simulink model "encode_decode_withAlarms_correction1"  (R2022a)
settings: Solver=VariableStepAuto  StartTime=0.0  StopTime=200  RelTol=1e-3
libraries: simulink x7, spsSampleandHoldLib x2
settings Model: Creator=mluser  LastModifiedBy=mluser
settings ModelReferenceCC: EnableRefExpFcnMdlSchedulingChecks=off
settings RTWCC: Description=Generic Real-Time Target

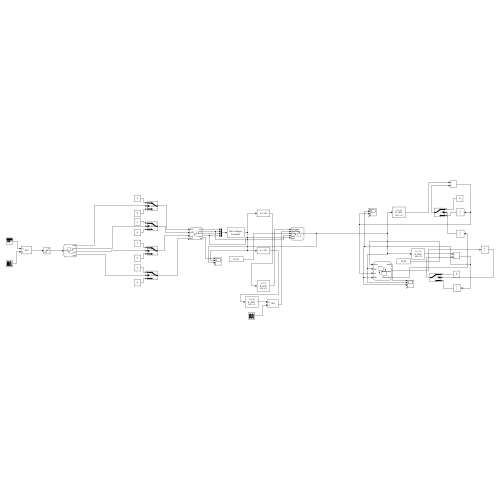
[thumbnail: Simulink's stored preview of the top-level diagram]
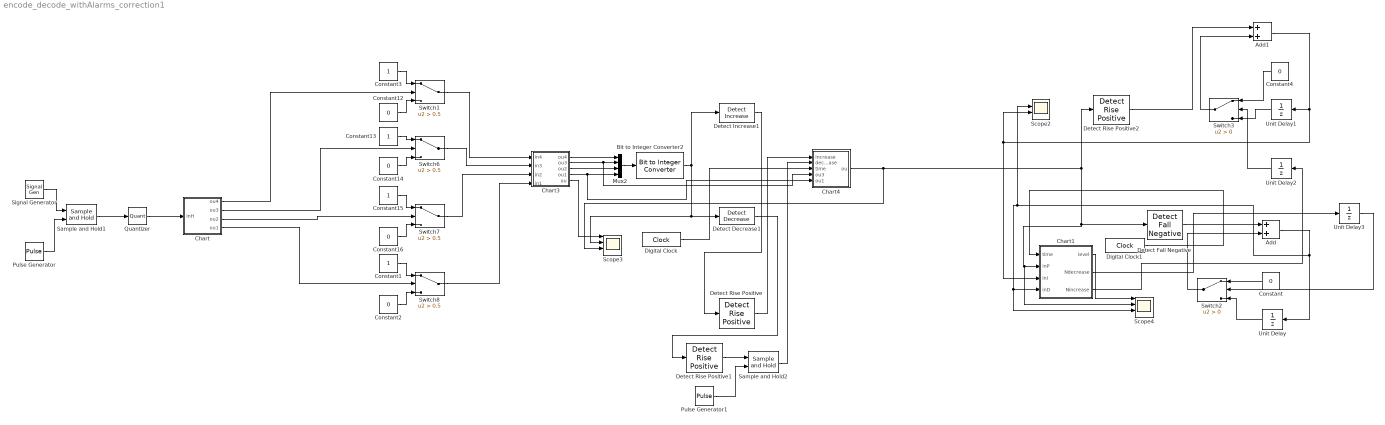
== system encode_decode_withAlarms_correction1 ==
  Add : Sum
  Add1 : Sum
  Bit to Integer Converter2 : simulink/Logic and Bit Operations/Bit to Integer Converter  nbits=4  bitOrder=MSB first  signedOutputValues=Unsigned  outDtype=Inherit via internal rule  outDtypeSigned=Inherit via internal rule
  Chart : Stateflow chart  TreatAsAtomicUnit=on
      settings: PortSchema="{\"entries\":[{\"content\":{\"sides\":[{\"content\":{\"connectorIds\":[\"In1\"]},\"type\":\"ConnectorPlacement.EquallySpacedRectSide\",\"uuid\":\"aaeedc4a-65ef-4d8f-ba01-1ddc4e011816\"},{\"content\":{\"connectorIds\":[\"Out2\",\"Out1\",\"Out3\",\"Out4\"],\"side\":\"RIGHT\"},\"type\":\"ConnectorPlacement.EquallySpacedRectSide\",\"uuid\":\"bfc75945-f598-4b29-99c0-df6bb3f156b5\"},{\"content\":{\"connectorIds\":[],\"side\":\"TOP\"},\"type\":\"ConnectorPlacement.EquallySpacedRectSide\",\"uuid\":\"e78d9c07-753c-4a5b-aa63-095c584c660c\"}]},\"type\":\"ConnectorPlacement.EquallySpacedConnector\",\"uuid\":\"f46ef6be-e67f-4bb7-838b-d108f8d3e6f5\"}],\"packageUris\":[\"http://schema.mathworks.com/mf0/Connector/R2020b\"],\"version\":\"1.0\"}"
  Chart1 : Stateflow chart  TreatAsAtomicUnit=on
  Chart3 : Stateflow chart  TreatAsAtomicUnit=on
      settings: PortSchema="{\"entries\":[{\"content\":{\"sides\":[{\"content\":{\"connectorIds\":[\"In3\",\"In2\",\"In1\",\"In4\"]},\"type\":\"ConnectorPlacement.EquallySpacedRectSide\",\"uuid\":\"6156c126-4374-4c11-ab2d-af131cd3e62a\"},{\"content\":{\"connectorIds\":[\"Out4\",\"Out3\",\"Out1\",\"Out5\",\"Out2\"],\"side\":\"RIGHT\"},\"type\":\"ConnectorPlacement.EquallySpacedRectSide\",\"uuid\":\"cbc23dfa-74ba-4e75-ac9f-4e20cfd8edcb\"},{\"content\":{\"connectorIds\":[],\"side\":\"TOP\"},\"type\":\"ConnectorPlacement.EquallySpacedRectSide\",\"uuid\":\"6ff231dc-a29b-42f5-ba4f-c5284aabb986\"}]},\"type\":\"ConnectorPlacement.EquallySpacedConnector\",\"uuid\":\"9e5f2232-d3ec-4fcd-9ee4-7d051677f9b4\"}],\"packageUris\":[\"http://schema.mathworks.com/mf0/Connector/R2020b\"],\"version\":\"1.0\"}"
  Chart4 : Stateflow chart  TreatAsAtomicUnit=on
  Constant{,2,4,12,14,16} (6 alike) : Constant  Value=0
  Constant{1,3,13,15} (4 alike) : Constant
  Detect Decrease1 : simulink/Logic and Bit Operations/Detect Decrease  vinit=0.0  OutDataTypeStr=boolean
  Detect Increase1 : simulink/Logic and Bit Operations/Detect Increase  vinit=0.0  OutDataTypeStr=boolean
  Detect Fall Negative : simulink/Logic and Bit Operations/Detect Fall Negative  vinit=0  OutDataTypeStr=boolean
  Detect Rise Positive : simulink/Logic and Bit Operations/Detect Rise Positive  vinit=0  OutDataTypeStr=boolean
  Detect Rise Positive1 : simulink/Logic and Bit Operations/Detect Rise Positive  vinit=0  OutDataTypeStr=boolean
  Detect Rise Positive2 : simulink/Logic and Bit Operations/Detect Rise Positive  vinit=0  OutDataTypeStr=boolean
  Digital Clock : DigitalClock  SampleTime=0.01
  Digital Clock1 : DigitalClock  SampleTime=0.01
  Mux2 : Mux
  Pulse Generator : DiscretePulseGenerator  PulseType=Time based  Period=0.01  PulseWidth=5  PhaseDelay=0.1
  Pulse Generator1 : DiscretePulseGenerator  PulseType=Time based  Period=0.01  PulseWidth=5
  Quantizer : Quantizer
  Sample and Hold1 : spsSampleandHoldLib/Sample and Hold  ic=0  Ts=0.1
  Sample and Hold2 : spsSampleandHoldLib/Sample and Hold  ic=0  Ts=0.01
  Scope2 : Scope  NumInputPorts=4
  Scope3 : Scope  NumInputPorts=4
  Scope4 : Scope  NumInputPorts=4
  Signal Generator : SignalGenerator  Amplitude=40  Frequency=0.02  Units=rad/sec
  Switch{1,6..8} (4 alike) : Switch  Criteria=u2 > Threshold  Threshold=0.5  SaturateOnIntegerOverflow=off  InputSameDT=off
  Switch2 : Switch  Criteria=u2 > Threshold  SaturateOnIntegerOverflow=off  InputSameDT=off
  Switch3 : Switch  Criteria=u2 > Threshold  SaturateOnIntegerOverflow=off  InputSameDT=off
  Unit Delay{,1..3} (4 alike) : UnitDelay  SampleTime=-1  HasFrameUpgradeWarning=on
  wires:
  Constant4/1 -> Switch3/1
  Sample and Hold1/1 -> Quantizer/1
  Switch1/1 -> Chart3/3(in4)
  Unit Delay2/1 -> Switch3/2
  Chart4/1(ou) -> Scope3/3, Scope4/2, Chart1/2(inP), Detect Fall Negative/1, Detect Rise Positive2/1
  Constant3/1 -> Switch1/1
  Add1/1 -> Chart1/3(inI), Scope2/3, Unit Delay1/1
  Constant15/1 -> Switch7/1
  Switch3/1 -> Add1/2
  Constant14/1 -> Switch6/3
  Constant1/1 -> Switch8/1
  Constant/1 -> Switch2/1
  Unit Delay3/1 -> Switch2/2
  Unit Delay/1 -> Switch2/3
  Digital Clock1/1 -> Chart1/1(time)
  Chart/3(ou2) -> Switch7/2
  Pulse Generator/1 -> Sample and Hold1/2
  Signal Generator/1 -> Sample and Hold1/1
  Unit Delay1/1 -> Switch3/3
  Constant13/1 -> Switch6/1
  Chart/1(ou3) -> Switch6/2
  Constant12/1 -> Switch1/3
  Constant16/1 -> Switch7/3
  Detect Fall Negative/1 -> Add/1
  Switch2/1 -> Add/2
  Chart/4(ou1) -> Switch8/2
  Chart/2(ou4) -> Switch1/2
  Switch8/1 -> Chart3/4(in1)
  Quantizer/1 -> Chart/1(inH)
  Constant2/1 -> Switch8/3
  Detect Rise Positive2/1 -> Add1/1
  Switch6/1 -> Chart3/2(in3)
  Switch7/1 -> Chart3/1(in2)
  Chart3/4(ou4) -> Mux2/1
  Chart3/1(ou2) -> Mux2/3
  Chart3/3(ou3) -> Chart4/4(ou3), Mux2/2
  Detect Rise Positive/1 -> Chart4/1(increase)
  Detect Decrease1/1 -> Detect Rise Positive1/1
  Chart3/5(ou1) -> Chart4/5(ou1), Mux2/4
  Detect Increase1/1 -> Detect Rise Positive/1
  Sample and Hold2/1 -> Chart4/2(decrease)
  Digital Clock/1 -> Chart4/3(time)
  Detect Rise Positive1/1 -> Sample and Hold2/1
  Pulse Generator1/1 -> Sample and Hold2/2
  Chart3/2(ou) -> Scope3/1
  Mux2/1 -> Bit to Integer Converter2/1
  Chart1/2(Ndecrease) -> Unit Delay3/1
  Chart1/3(Nincrease) -> Unit Delay2/1
  Chart1/1(level) -> Scope4/1
  Add/1 -> Unit Delay/1, Scope4/3, Chart1/4(inD), Scope2/2
  Bit to Integer Converter2/1 -> Scope3/2, Detect Decrease1/1, Detect Increase1/1

== stateflow chart encode_decode_withAlarms_correction1/Chart ==
  (default) -> (junction 3) : {ou1=0;
      | ou2=0;
      | ou3=0;
      | ou4=0;
      | }
  (junction 3) -> (junction 28) [order 2] : [inH==0]
  (junction 28) -> (junction 44) : {ou1=0;ou2=0;ou3=0;ou4=0;}
  (junction 3) -> (junction 10) [order 1]
  (junction 44) -> (junction 43)
  (junction 10) -> (junction 8) [order 1] : [inH<=10]
  (junction 8) -> (junction 43) : {ou1=1;ou2=0;ou3=0;ou4=0;}
  (junction 10) -> (junction 12) [order 2]
  (junction 43) -> (junction 42)
  (junction 16) -> (junction 42) : {ou1=1;ou2=1;ou3=0;ou4=0;}
  (junction 12) -> (junction 16) [order 1] : [inH>10&&inH<=20]
  (junction 42) -> (junction 41)
  (junction 12) -> (junction 19) [order 2]
  (junction 19) -> (junction 18) [order 1] : [inH>20&&inH<=30]
  (junction 18) -> (junction 41) : {ou1=1;ou2=1;ou3=1;ou4=0;}
  (junction 41) -> (junction 63)
  (junction 19) -> (junction 61) [order 2]
  (junction 61) -> (junction 62) : [inH>30]
  (junction 62) -> (junction 63) : {ou1=1;ou2=1;ou3=1;ou4=1;}
  data: ou3 output; ou4 output; ou2 output; ou1 output; inH input

== stateflow chart encode_decode_withAlarms_correction1/Chart3 ==
  state q1
    entry:ou1=0;ou2=0;
    ou3=0;ou4=0;
  state q2
    entry:ou1=1;ou2=0;
    ou3=0;ou4=0;
  state Input
    entry:
  state q3
    entry:ou1=1;ou2=1;
    ou3=0;ou4=0;
  state q4
    entry:ou1=1;ou2=1;
    ou3=1;ou4=0;
  state q5
    entry:ou1=1;ou2=1;
    ou3=1;ou4=1;
  Input -> q1 [order 1] : [in1==1&&in2==0&&in3==0&&in4==0]
      | {ou=0;}
  q1 -> q2 : [in1==1&&in2==0&&in3==0&&in4==0]
      | {ou=1;}
  q2 -> q1 [order 1] : [in1==0&&in2==0&&in3==0&&in4==0]
      | {ou=0;}
  q2 -> q3 [order 2] : [in1==1&&in2==1&&in3==0&&in4==0]
      | {ou=1;}
  q3 -> q2 [order 1] : [in1==1&&in2==0&&in3==0&&in4==0]
      | {ou=0;}
  (default) -> Input
  Input -> q5 [order 2] : [in1==1&&in2==1&&in3==1&&in4==1]
      | {ou=1;}
  q3 -> q4 [order 2] : [in1==1&&in2==1&&in3==1&&in4==0]
      | {ou=1;}
  q4 -> q3 [order 1] : [in1==1&&in2==1&&in3==0&&in4==0]
      | {ou=0;}
  q4 -> q5 [order 2] : [in1==1&&in2==1&&in3==1&&in4==1]
      | {ou=1;}
  q5 -> q4 : [in1==1&&in2==1&&in3==1&&in4==0]
      | {ou=0;}
  data: in2 input; in3 input; in4 input; in1 input; ou2 output; ou output; ou3 output; ou4 output; ou1 output

== stateflow chart encode_decode_withAlarms_correction1/Chart4 ==
  (default) -> (junction 3)
  (junction 3) -> (junction 28) [order 2] : [increase==1&&time>0]
  (junction 28) -> (junction 44) : {ou=1;}
  (junction 3) -> (junction 10) [order 1]
  (junction 44) -> (junction 43)
  (junction 10) -> (junction 8) [order 1] : [decrease==1&&time>0]
  (junction 8) -> (junction 43) : {ou=-1;}
  (junction 10) -> (junction 71) [order 2]
  (junction 43) -> (junction 72)
  (junction 71) -> (junction 73) [order 1] : [time==0&&ou3==1]
  (junction 73) -> (junction 72) : {ou=1;}
  (junction 71) -> (junction 78) [order 2]
  (junction 72) -> (junction 80)
  (junction 78) -> (junction 79) [order 1] : [time==0&&ou1==0]
  (junction 79) -> (junction 80) : {ou=-1;}
  (junction 78) -> (junction 90) [order 2]
  (junction 80) -> (junction 88)
  (junction 89) -> (junction 88) : {ou=0}
  (junction 90) -> (junction 89) : [increase==0&&decrease==0]
  data: increase input; decrease input; ou output; time input; ou3 input; ou1 input

== stateflow chart encode_decode_withAlarms_correction1/Chart1 ==
  state state1
    entry:
    level=0;
    Ndecrease=0;
    Nincrease=0;
  state initial
    entry:
    Ndecrease=0;
    Nincrease=0;
  state state2
    entry:
    level=1;
    Ndecrease=0;
    Nincrease=0;
  state state3
    entry:
    level=2;
    Ndecrease=0;
    Nincrease=0;
  state state5
    entry:
    level=4;
    Ndecrease=0;
    Nincrease=0;
  state state4
    entry:
    level=3;
    Nincrease=0;
    Ndecrease=0;
  (default) -> initial
  state1 -> state2 : [time>=1&&inP==1&&inI==1]
  initial -> state1 [order 2] : [time<1&&inP==1]
      | {Ndecrease=0;
      | Nincrease=0;}
  (junction 29) -> state1 : {Ndecrease=1;
      | Nincrease=1;}
  initial -> state5 [order 1] : [time<1&&inP==-1]
  state2 -> (junction 29) [order 2] : [time>=1&&inP==-1&&inD==5]
  state3 -> state2 [order 2] : [time>=1&&inP==-1&&inD==4]
  state2 -> state3 [order 1] : [time>=1&&inP==1&&inI==1]
  state3 -> state4 [order 1] : [time>=1&&inP==1&&inI==2]
  state4 -> state3 [order 2] : [time>=1&&inP==-1&&inD==3]
  state4 -> (junction 30) [order 1] : [time>=1&&inP==1&&inI==2]
  (junction 30) -> state5 : {Ndecrease=1;
      | Nincrease=1;}
  state5 -> state4 : [time>=1&&inP==-1&&inD==2]
  data: time input; inP input; inI input; inD input; level output; Ndecrease output; Nincrease output
